simulink model "Fig349"  (R2014b)
settings: Solver=ode3  StartTime=0.0  StopTime=10.002  FixedStep=2e-6  RelTol=1e-5
libraries: dsparch4 x2, commchan3 x1, commsink2 x1, commrandsrc2 x1
settings Model: Creator=Dennis Silage  LastModifiedBy=Silage
settings DataIOCC: SignalLoggingSaveFormat=ModelDataLogs
settings OptimizationCC: ExpressionDepthLimit=2147483647  InitFltsAndDblsToZero=on
settings DebuggingCC: UnderspecifiedInitializationDetection=Classic  MergeDetectMultiDrivingBlocksExec=none  SolverPrmCheckMsg=none  FcnCallInpInsideContextMsg=UseLocalSettings  StateNameClashWarn=warning
settings GRTTargetCC: CombineOutputUpdateFcns=off  GRTInterface=on

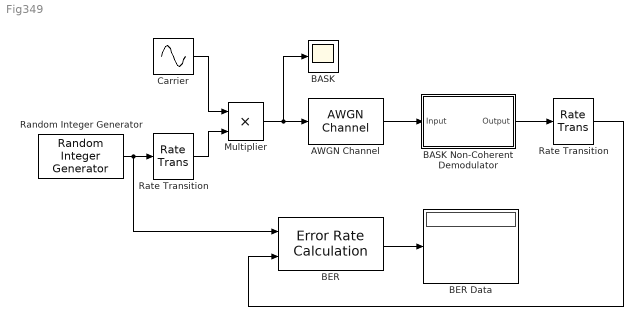
== system Fig349 ==
  AWGN Channel : commchan3/AWGN Channel  InputProcessing=Inherited (this choice will be removed - see release notes)  seed=randseed  noiseMode="Signal to noise ratio  (Eb/No)"  EbNodB=16  EsNodB=10  SNRdB=12  bitsPerSym=1  Ps=12.5  Tsym=1e-3  variance=0
  BASK : Scope
      settings: YMin=-6  YMax=6
  BASK Non-Coherent Demodulator : Subsystem
  BER : commsink2/Error Rate Calculation  N=3  st_delay=0  cp_mode=Entire frame  subframe=[]  PMode=Port  WsName=ErrorVec  RsMode2=off  stop=off  numErr=100  maxBits=1e6
  BER Data : Display
  Carrier : Sin  Amplitude=5  Frequency=40000*pi  SampleTime=2e-6
  "Multiplier " : Product  RndMeth=Zero
  Random Integer Generator : commrandsrc2/Random Integer Generator  mul=2  seed=randseed  Ts=1e-3  frameBased=off  sampPerFrame=50  orient=on  outDataType=double
  "Rate Transition  " : RateTransition  OutPortSampleTime=1e-3
  Rate Transition : RateTransition  OutPortSampleTime=2e-6
  wires:
  Random Integer Generator/1 -> Rate Transition/1, BER/1
  BER/1 -> BER Data/1
  "Multiplier "/1 -> AWGN Channel/1, BASK/1
  Carrier/1 -> "Multiplier "/1
  Rate Transition/1 -> "Multiplier "/2
  AWGN Channel/1 -> BASK Non-Coherent Demodulator/1(Input)
  BASK Non-Coherent Demodulator/1(Output) -> "Rate Transition  "/1
  "Rate Transition  "/1 -> BER/2

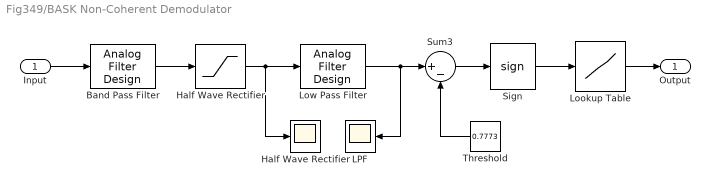
== system Fig349/BASK Non-Coherent Demodulator ==
  Input : Inport
  Band Pass Filter : dsparch4/Analog Filter Design  method=Butterworth  filttype=Bandpass  N=9  Wlo=38000*pi  Whi=42000*pi  Rp=2  Rs=40
  Half Wave Rectifier : Saturate  UpperLimit=2000  LowerLimit=0
  "Half Wave Rectifier " : Scope
      settings: YMin=-0.5  YMax=6
  LPF : Scope
      settings: YMin=-0.5  YMax=2  SaveName=ScopeData2
  Lookup Table : Lookup_n-D  NumberOfTableDimensions=1  BreakpointsForDimension1=[-1, 0, 1]  Table=[0, 0, 1]  InternalRulePriority=Speed  RndMeth=Simplest  InputSameDT=on
  Low Pass Filter : dsparch4/Analog Filter Design  method=Butterworth  filttype=Lowpass  N=9  Wlo=4000*pi  Whi=46000*pi  Rp=2  Rs=40
  Sign : Signum
  Sum3 : Sum  Inputs=|+-
  Threshold : Constant  Value=0.7773
  Output : Outport
  wires:
  Sign/1 -> Lookup Table/1
  Input/1 -> Band Pass Filter/1
  Band Pass Filter/1 -> Half Wave Rectifier/1
  Lookup Table/1 -> Output/1
  Half Wave Rectifier/1 -> Low Pass Filter/1, "Half Wave Rectifier "/1
  Low Pass Filter/1 -> Sum3/1, LPF/1
  Sum3/1 -> Sign/1
  Threshold/1 -> Sum3/2
